simulink library "mtq_lib_dc2m"  (R2018b)
settings: Solver=VariableStepAuto  StartTime=0.0  StopTime=10.0  RelTol=1e-3
undefined symbols (not defined in the file): fswParams, simParams
settings Model: Creator=Taylor  LastModifiedBy=colem

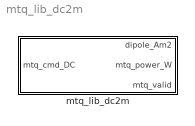
== system mtq_lib_dc2m ==
  mtq_lib_dc2m : Subsystem

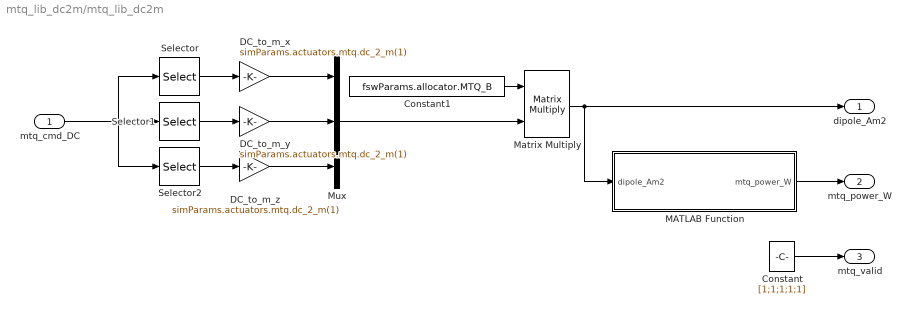
== system mtq_lib_dc2m/mtq_lib_dc2m ==
  mtq_cmd_DC : Inport
  Constant : Constant  Value=[1;1;1;1;1]  SampleTime=simParams.sample_time_s
  Constant1 : Constant  Value=fswParams.allocator.MTQ_B  SampleTime=simParams.sample_time_s
  DC_to_m_x : Gain  Gain=simParams.actuators.mtq.dc_2_m(1)
  DC_to_m_y : Gain  Gain=simParams.actuators.mtq.dc_2_m(1)
  DC_to_m_z : Gain  Gain=simParams.actuators.mtq.dc_2_m(1)
  MATLAB Function : MATLAB Function  TreatAsAtomicUnit=on
  Matrix Multiply : Product  Multiplication=Matrix(*)
  Mux : Mux  Inputs=[2 2 1]
  Selector : Selector  InputPortWidth=sum(simParams.actuators.mtq.n_coils)  IndexOptions=Index vector (dialog)  Indices=simParams.actuators.mtq.id_x  OutputSizes=1
  Selector1 : Selector  InputPortWidth=sum(simParams.actuators.mtq.n_coils)  IndexOptions=Index vector (dialog)  Indices=simParams.actuators.mtq.id_y  OutputSizes=1
  Selector2 : Selector  InputPortWidth=sum(simParams.actuators.mtq.n_coils)  IndexOptions=Index vector (dialog)  Indices=simParams.actuators.mtq.id_z  OutputSizes=1
  dipole_Am2 : Outport
  mtq_power_W : Outport  Port=2
  mtq_valid : Outport  Port=3
  wires:
  MATLAB Function/1(mtq_power_W) -> mtq_power_W/1
  mtq_cmd_DC/1 -> Selector2/1, Selector/1, Selector1/1
  Selector/1 -> DC_to_m_x/1
  Selector2/1 -> DC_to_m_z/1
  Selector1/1 -> DC_to_m_y/1
  DC_to_m_x/1 -> Mux/1
  DC_to_m_z/1 -> Mux/3
  DC_to_m_y/1 -> Mux/2
  Constant/1 -> mtq_valid/1
  Constant1/1 -> Matrix Multiply/1
  Matrix Multiply/1 -> MATLAB Function/1("dipole_Am2 "), dipole_Am2/1
  Mux/1 -> Matrix Multiply/2

== matlab function mtq_lib_dc2m/MATLAB Function ==
  data: dipole_Am2 input; mtq_power_W output; simParams parameter
function mtq_power_W  = mtq_power(dipole_Am2,simParams)
% Maps the MTQ dipole to power using a linear relationship assuming that
% they consume P_max when commanded to dipole m_max, and zero power for
% zero dipole. 
%
% Evenly distributes the dipole to any body axes that have
% multiple coils. Outputs total power only in Watts.
%
% T. Reynolds
%#codegen

n_coils = simParams.actuators.mtq.n_coils;
id_x    = simParams.actuators.mtq.id_x;
id_y    = simParams.actuators.mtq.id_y;
id_z    = simParams.actuators.mtq.id_z;
m_to_P  = simParams.actuators.mtq.dipole_to_power;

coil_dipole = zeros(sum(n_coils),1);
coil_power  = zeros(sum(n_coils),1);

coil_dipole(id_x) = dipole_Am2(1)/n_coils(1);
coil_dipole(id_y) = dipole_Am2(2)/n_coils(2);
coil_dipole(id_z) = dipole_Am2(3)/n_coils(3);

coil_power(id_x) = abs(coil_dipole(id_x)) .* m_to_P(1);
coil_power(id_y) = abs(coil_dipole(id_y)) .* m_to_P(2);
coil_power(id_z) = abs(coil_dipole(id_z)) .* m_to_P(3);

mtq_power_W = sum(coil_power);

end
